simulink model "LAVM_torque"  (R2022b)
settings: Solver=FixedStepDiscrete  StartTime=0.0  StopTime=3  FixedStep=Tsim  MaxStep=Tsim  RelTol=1e-7
values from neighbouring files (symbols this model uses):
  flux = 0.025    [LAVM_torque.sldd]
  J = 4.982E-8    [LAVM_torque.sldd]
  ka = 0.027    [LAVM_torque.sldd]
  kc = 0.008    [LAVM_torque.sldd]
  L_com = 0.00094    [LAVM_torque.sldd]
  L_dif = 6.0E-5    [LAVM_torque.sldd]
  R = 4.27    [LAVM_torque.sldd]
  Tsim = 1.0E-6    [LAVM_torque.sldd]
undefined symbols (not defined in the file or in its folder): DiscIntNeverNeededParam
libraries: dspstat3 x2, spsControlledVoltageSourceLib x1, spsControlledCurrentSourceLib x1, spsVoltageMeasurementLib x1, spspowerguiLib x1
settings Model: DataDictionary=LAVM_torque.sldd  Creator=SSC  LastModifiedBy=SSC
settings DataIOCC: ReturnWorkspaceOutputs=off

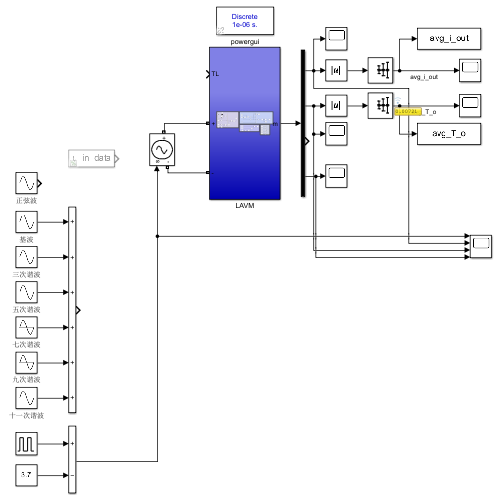
[thumbnail: Simulink's stored preview of the top-level diagram]
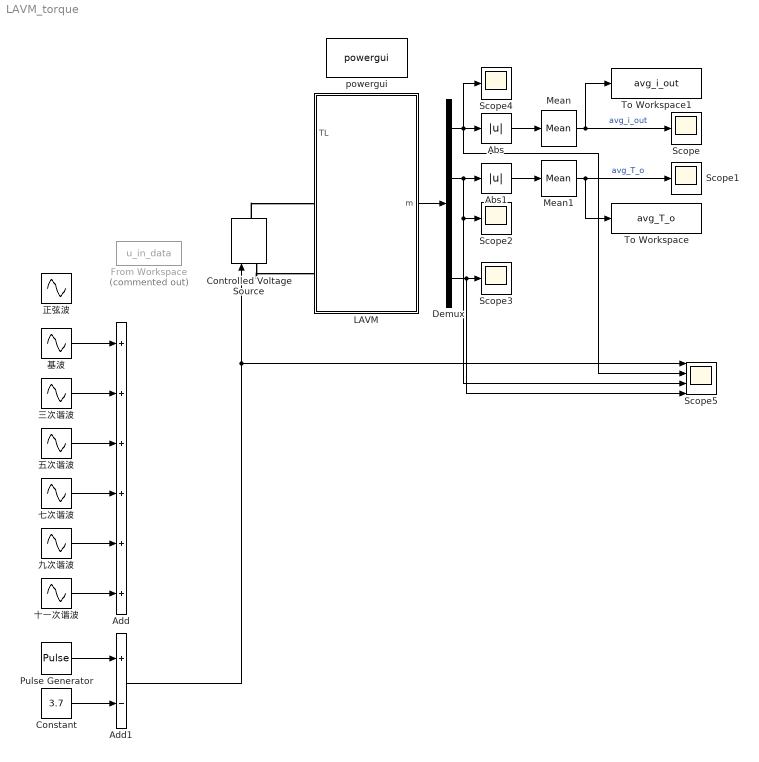
== system LAVM_torque ==
  Abs : Abs  SaturateOnIntegerOverflow=off
  Abs1 : Abs  SaturateOnIntegerOverflow=off
  Add : Sum  Inputs=++++++
  Add1 : Sum  Inputs=+-
  Constant : Constant  Value=3.7
  Controlled Voltage Source : spsControlledVoltageSourceLib/Controlled Voltage Source  Initialize=on  Source_Type=DC  Amplitude=0  Phase=0  Frequency=0  Measurements=None
  Demux : Demux
  From Workspace : FromWorkspace  Commented=on  VariableName=u_in_data  SampleTime=Tsim
  LAVM : Subsystem
  Mean : dspstat3/Mean  run=on  InputProcessing=Columns as channels (frame based)  reset_popup=None  directionMode=Each column  dimension=1  roiEnable=off  roiType=Rectangles  roiPortion=Entire ROI  roiOutput=Individual statistics for each ROI  roiFlag=off  roundingMode=Floor  overflowMode=off  outputDataTypeStr=Inherit: Same as accumulator  outputMin=[]  outputMax=[]  outputLastDataTypeStr=Inherit: Same as accumulator
  Mean1 : dspstat3/Mean  run=on  InputProcessing=Columns as channels (frame based)  reset_popup=None  directionMode=Each column  dimension=1  roiEnable=off  roiType=Rectangles  roiPortion=Entire ROI  roiOutput=Individual statistics for each ROI  roiFlag=off  roundingMode=Floor  overflowMode=off  outputDataTypeStr=Inherit: Same as accumulator  outputMin=[]  outputMax=[]  outputLastDataTypeStr=Inherit: Same as accumulator
  Pulse Generator : DiscretePulseGenerator  PulseType=Time based  Amplitude=3.7*2  Period=1/200  PulseWidth=50
  Scope{,1..4} (5 alike) : Scope
  Scope5 : Scope  NumInputPorts=4
  To Workspace : ToWorkspace  VariableName=avg_T_o  SampleTime=-1
      settings: MaxDataPoints=1  Save2DSignal=2-D array (concatenate along first dimension)
  To Workspace1 : ToWorkspace  VariableName=avg_i_out  SampleTime=-1
      settings: MaxDataPoints=1  Save2DSignal=2-D array (concatenate along first dimension)
  powergui : spspowerguiLib/powergui  Priority=1  SimulationMode=Discrete  SampleTime=Tsim  frequency=60  Iterations=50  frequencyindice=0  Pbase=100e6  ErrMax=1e-4  UnitsV=kV  UnitsW=MW  buscounter=0  FunctionMessages=off  echomessages=off  EnableUseOfTLC=off  CurrentSourceSwitches=off  DisableSnubberDevices=off  DisableRonSwitches=off  DisableVfSwitches=off  DisplayEquations=off  AutomaticDiscreteSolvers=off  SolverType=Tustin/Backward Euler (TBE)  Interpol=off  ExternalGateDelay=off  methode=off  Ts=100  x0status=blocks  SPID=on  SwTol=0  HookPort=off  NonlinearTolerance=1e-4  nMaxIteration=100  ContinueOnMaxIteration=off  RestoreLinks=warning  ResistiveCurrentMeasurement=off  Frange=[0:2:500]  Ylog=off  Xlog=on  ShowGrid=off  save=off  variable=ZData  structure=0  ZoomFFT=off  StartTime=0.0  cycles=1  DisplayStyle=1  fundamental=60  FreqAxis=off  MaxFrequency=1000  frequencyindicesteady=1  RmsSteady=1  display=off
  七次谐波 : Sin  Amplitude=0.93  Frequency=242*2*pi*7  SampleTime=0
  三次谐波 : Sin  Amplitude=2.35  Frequency=242*2*pi*3  SampleTime=0
  九次谐波 : Sin  Amplitude=-0.04  Frequency=242*2*pi*9  SampleTime=0
  五次谐波 : Sin  Amplitude=-0.01  Frequency=242*2*pi*5  SampleTime=0
  十一次谐波 : Sin  Amplitude=0.25  Frequency=242*2*pi*11  SampleTime=0
  基波 : Sin  Amplitude=3.58  Frequency=242*2*pi  SampleTime=0
  正弦波 : Sin  Amplitude=3.7  Frequency=280*2*pi  SampleTime=0
  wires:
  LAVM/1(m) -> Demux/1
  Demux/1 -> Scope4/1, Scope5/2, Abs/1
  Abs/1 -> Mean/1
  Mean/1 -> To Workspace1/1, Scope/1  "avg_i_out"
  Demux/2 -> Scope5/3, Scope2/1, Abs1/1
  Abs1/1 -> Mean1/1
  基波/1 -> Add/1
  三次谐波/1 -> Add/2
  五次谐波/1 -> Add/3
  七次谐波/1 -> Add/4
  九次谐波/1 -> Add/5
  十一次谐波/1 -> Add/6
  Demux/4 -> Scope5/4, Scope3/1
  Mean1/1 -> To Workspace/1, Scope1/1  "avg_T_o"
  Pulse Generator/1 -> Add1/1
  Constant/1 -> Add1/2
  Add1/1 -> Controlled Voltage Source/1, Scope5/1
  connections:
  Controlled Voltage Source/RConn1 -- LAVM/LConn1
  Controlled Voltage Source/LConn1 -- LAVM/LConn2

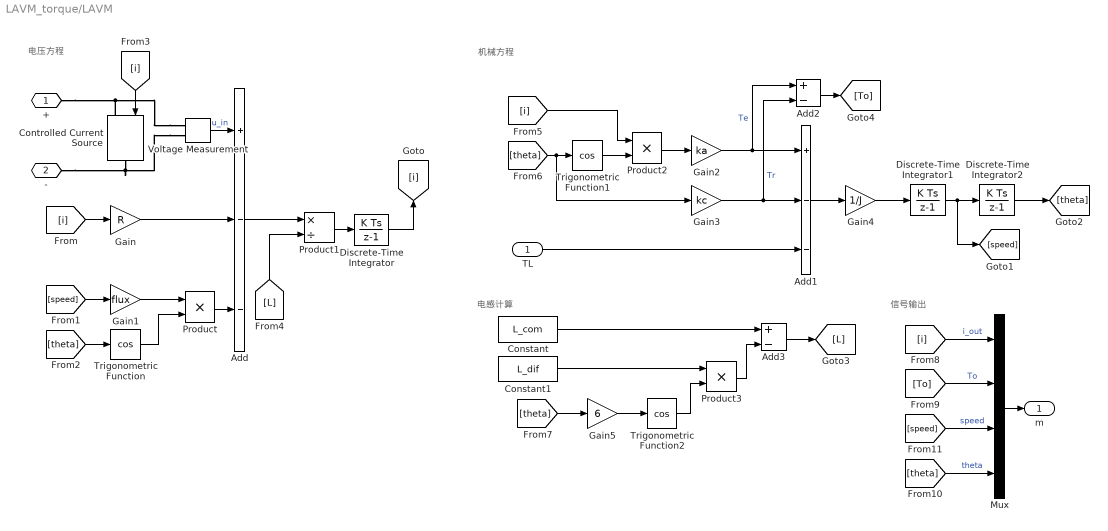
== system LAVM_torque/LAVM ==
  note: 信号输出
  note: 电感计算
  note: 机械方程
  note: 电压方程
  TL : Inport
  Add : Sum  Inputs=+--
  Add1 : Sum  Inputs=+--
  Add2 : Sum  Inputs=+-
  Add3 : Sum  Inputs=+-
  Constant : Constant  Value=L_com
  Constant1 : Constant  Value=L_dif
  Controlled Current Source : spsControlledCurrentSourceLib/Controlled Current Source  Initialize=on  Source_Type=AC  Amplitude=0  Phase=0  Frequency=0  Measurements=None
  Discrete-Time Integrator : DiscreteIntegrator  SampleTime=-1  ICPrevOutput=DiscIntNeverNeededParam  ICPrevScaledInput=DiscIntNeverNeededParam
  Discrete-Time Integrator1 : DiscreteIntegrator  SampleTime=-1  ICPrevOutput=DiscIntNeverNeededParam  ICPrevScaledInput=DiscIntNeverNeededParam
  Discrete-Time Integrator2 : DiscreteIntegrator  SampleTime=-1  ICPrevOutput=DiscIntNeverNeededParam  ICPrevScaledInput=DiscIntNeverNeededParam
  Gain : Gain  Gain=R
  Gain1 : Gain  Gain=flux
  Gain2 : Gain  Gain=ka
  Gain3 : Gain  Gain=kc
  Gain4 : Gain  Gain=1/J
  Gain5 : Gain  Gain=6
  Mux : Mux
  Product : Product
  Product1 : Product  Inputs=*/
  Product2 : Product
  Product3 : Product
  Trigonometric Function : Trigonometry  Operator=cos
  Trigonometric Function1 : Trigonometry  Operator=cos
  Trigonometric Function2 : Trigonometry  Operator=cos
  Voltage Measurement : spsVoltageMeasurementLib/Voltage Measurement  PhasorSimulation=off  OutputType=Complex  PSBequivalent=0
  + : PMIOPort  Side=Left
  - : PMIOPort  Port=2  Side=Left
  m : Outport
  wires:
  Product1/1 -> Discrete-Time Integrator/1
  [speed] -> Gain1/1
  [i] -> Controlled Current Source/1
  [L] -> Product1/2
  Add/1 -> Product1/1
  Discrete-Time Integrator/1 -> [i]
  [i] -> Gain/1
  Product/1 -> Add/3
  Gain/1 -> Add/2
  Trigonometric Function/1 -> Product/2
  Gain1/1 -> Product/1
  [theta] -> Trigonometric Function/1
  Voltage Measurement/1 -> Add/1  "u_in"
  [theta] -> Gain3/1, Trigonometric Function1/1
  [i] -> Product2/1
  Trigonometric Function1/1 -> Product2/2
  Product2/1 -> Gain2/1
  Gain2/1 -> Add2/1, Add1/1  "Te"
  Gain3/1 -> Add2/2, Add1/2  "Tr"
  TL/1 -> Add1/3
  Add1/1 -> Gain4/1
  Gain4/1 -> Discrete-Time Integrator1/1
  Discrete-Time Integrator1/1 -> [speed], Discrete-Time Integrator2/1
  Discrete-Time Integrator2/1 -> [theta]
  Constant/1 -> Add3/1
  [theta] -> Gain5/1
  Gain5/1 -> Trigonometric Function2/1
  Trigonometric Function2/1 -> Product3/2
  Constant1/1 -> Product3/1
  Product3/1 -> Add3/2
  Add3/1 -> [L]
  [i] -> Mux/1  "i_out"
  Add2/1 -> [To]
  [theta] -> Mux/4  "theta"
  [speed] -> Mux/3  "speed"
  [To] -> Mux/2  "To"
  Mux/1 -> m/1
  connections:
  Voltage Measurement/LConn1 -- +/RConn1 -- Controlled Current Source/LConn1
  Voltage Measurement/LConn2 -- -/RConn1 -- Controlled Current Source/RConn1
